simulink subsystem "attitude_determination_and_vehicle_est"  (R2024a)
settings: Solver=VariableStepAuto  StartTime=0.0  StopTime=10.0  RelTol=1e-3
settings Model: Creator=joshu  LastModifiedBy=joshu

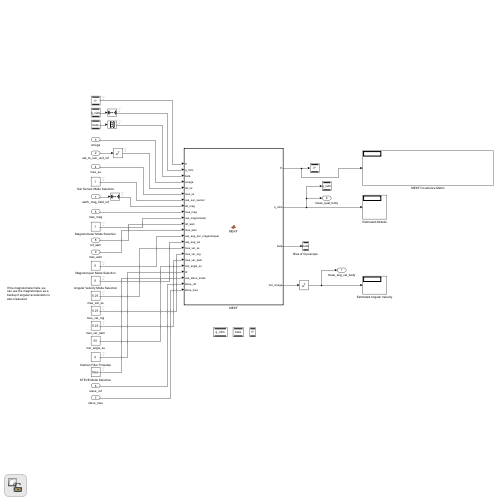
[thumbnail: Simulink's stored preview of the top-level diagram]
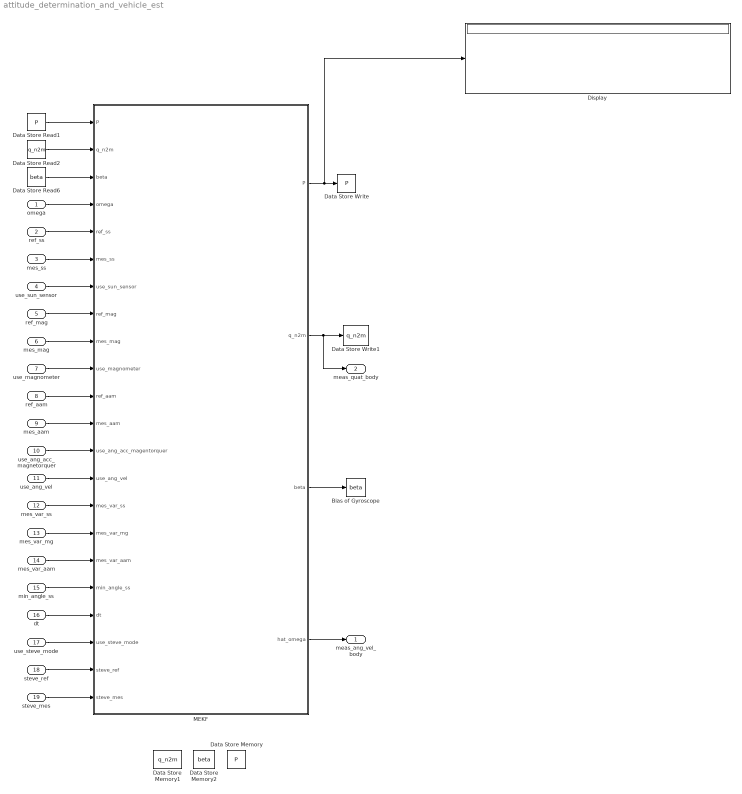
== system attitude_determination_and_vehicle_est ==
  omega : Inport
  ref_ss : Inport  Port=2
  mes_ss : Inport  Port=3
  use_sun_sensor : Inport  Port=4
  ref_mag : Inport  Port=5
  mes_mag : Inport  Port=6
  use_magnometer : Inport  Port=7
  ref_aam : Inport  Port=8
  mes_aam : Inport  Port=9
  use_ang_acc_magnetorquer : Inport  Port=10
  use_ang_vel : Inport  Port=11
  mes_var_ss : Inport  Port=12
  mes_var_mg : Inport  Port=13
  mes_var_aam : Inport  Port=14
  min_angle_ss : Inport  Port=15
  dt : Inport  Port=16
  use_steve_mode : Inport  Port=17
  steve_ref : Inport  Port=18
  steve_mes : Inport  Port=19
  Bias of Gyroscope : DataStoreWrite  DataStoreName=beta  IndexOptions=Index vector (dialog)  Indices=1  OutputSizes=1
  Data Store Memory : DataStoreMemory  DataStoreName=P  WriteAfterWriteMsg=warning  InitialValue=diag([1*ones(1,3), 1*ones(1,3)])  VectorParams1D=off  ShowAdditionalParam=off
      settings: LockScale=on
  Data Store Memory1 : DataStoreMemory  DataStoreName=q_n2m  WriteAfterWriteMsg=warning  InitialValue=q_n2m_initial  VectorParams1D=off  ShowAdditionalParam=off  Dimensions=[1,4]
  Data Store Memory2 : DataStoreMemory  DataStoreName=beta  WriteAfterWriteMsg=warning  InitialValue=beta_initial  VectorParams1D=off  ShowAdditionalParam=off  Dimensions=[1,3]
      settings: LockScale=on
  Data Store Read1 : DataStoreRead  DataStoreName=P  IndexOptions=Index vector (dialog)  Indices=1  OutputSizes=1
  Data Store Read2 : DataStoreRead  DataStoreName=q_n2m  IndexOptions=Index vector (dialog)  Indices=1  OutputSizes=1
  Data Store Read6 : DataStoreRead  DataStoreName=beta  IndexOptions=Index vector (dialog)  Indices=1  OutputSizes=1
  Data Store Write : DataStoreWrite  DataStoreName=P  IndexOptions=Index vector (dialog)  Indices=1  OutputSizes=1
  Data Store Write1 : DataStoreWrite  DataStoreName=q_n2m  IndexOptions=Index vector (dialog)  Indices=1  OutputSizes=1
  Display : Display
  MEKF : MATLAB Function  TreatAsAtomicUnit=on
  meas_ang_vel_body : Outport
  meas_quat_body : Outport  Port=2
  wires:
  MEKF/3(beta) -> Bias of Gyroscope/1
  MEKF/2(q_n2m) -> meas_quat_body/1, Data Store Write1/1
  MEKF/4(hat_omega) -> meas_ang_vel_body/1
  MEKF/1(P) -> Data Store Write/1, Display/1
  Data Store Read1/1 -> MEKF/1("P ")
  Data Store Read2/1 -> MEKF/2("q_n2m ")
  Data Store Read6/1 -> MEKF/3("beta ")
  omega/1 -> MEKF/4(omega)
  ref_ss/1 -> MEKF/5(ref_ss)
  mes_ss/1 -> MEKF/6(mes_ss)
  use_sun_sensor/1 -> MEKF/7(use_sun_sensor)
  ref_mag/1 -> MEKF/8(ref_mag)
  mes_mag/1 -> MEKF/9(mes_mag)
  use_magnometer/1 -> MEKF/10(use_magnometer)
  ref_aam/1 -> MEKF/11(ref_aam)
  mes_aam/1 -> MEKF/12(mes_aam)
  use_ang_acc_magnetorquer/1 -> MEKF/13(use_ang_acc_magentorquer)
  use_ang_vel/1 -> MEKF/14(use_ang_vel)
  mes_var_ss/1 -> MEKF/15(mes_var_ss)
  mes_var_mg/1 -> MEKF/16(mes_var_mg)
  mes_var_aam/1 -> MEKF/17(mes_var_aam)
  min_angle_ss/1 -> MEKF/18(min_angle_ss)
  dt/1 -> MEKF/19(dt)
  use_steve_mode/1 -> MEKF/20(use_steve_mode)
  steve_ref/1 -> MEKF/21(steve_ref)
  steve_mes/1 -> MEKF/22(steve_mes)

== matlab function attitude_determination_and_vehicle_est/MEKF ==
  data: P input size=[6, 6]; P output; q_n2m input size=[1,4]; beta input size=[1,3]; q_n2m output; beta output; omega input size=[1,3]; ref_ss input size=[1,3]; mes_ss input size=[1,3]; use_sun_sensor input boolean; ref_mag input; mes_mag input; use_magnometer input boolean; ref_aam input; mes_aam input; use_ang_acc_magentorquer input boolean; use_ang_vel input boolean; mes_var_ss input; mes_var_mg input; mes_var_aam input; min_angle_ss input; dt input; hat_omega output size=[1,3]; use_steve_mode input boolean; steve_ref input; steve_mes input
function [P, q_n2m,beta,hat_omega] = MEKF(P,q_n2m,beta,omega, ref_ss, mes_ss, use_sun_sensor, ref_mag, mes_mag, ...
                                            use_magnometer, ref_aam, mes_aam, use_ang_acc_magentorquer, use_ang_vel, ...
                                            mes_var_ss, mes_var_mg, mes_var_aam, min_angle_ss, dt, use_steve_mode, steve_ref, steve_mes)
    arguments (Input)
        P (6,6) double
        q_n2m (1,4) double
        beta (1,3) double
        omega (1,3) double
        ref_ss (1,3) double
        mes_ss (1,3) double
        use_sun_sensor (1,1) double %boolean
        ref_mag (1,3) double
        mes_mag (1,3) double
        use_magnometer (1,1) double %boolean
        ref_aam (1,3) double
        mes_aam (1,3) double
        use_ang_acc_magentorquer (1,1) double %boolean
        use_ang_vel (1,1) double %boolean
        mes_var_ss (1,1) double
        mes_var_mg (1,1) double
        mes_var_aam (1,1) double
        min_angle_ss (1,1) double
        dt  (1,1) double
        use_steve_mode  (1,1) double %boolean
        steve_ref (1,3) double
        steve_mes (1,3) double
    end

    arguments (Output)
        P (6,6) double
        q_n2m (1,4) double
        beta (1,3) double
        hat_omega (1,3) double
    end

    [P, q_n2m,beta,hat_omega] = fullMEKF(P, q_n2m, beta, omega, ref_ss, mes_ss, use_sun_sensor, ref_mag, mes_mag, ...
                                                use_magnometer, ref_aam, mes_aam, use_ang_acc_magentorquer, use_ang_vel, ...
                                                mes_var_ss, mes_var_mg, mes_var_aam, min_angle_ss, dt, use_steve_mode, steve_ref, steve_mes);
    
end
